simulink model "V2V"  (R2021a)
settings: Solver=FixedStepDiscrete  StartTime=0.0  StopTime=10  FixedStep=0.001  RelTol=1e-3
settings Model: Creator=maurizio  LastModifiedBy=maurizio
settings SolverCC: MinimalZcImpactIntegration=on
settings DebuggingCC: ReadBeforeWriteMsg=DisableAll  WriteAfterWriteMsg=DisableAll  WriteAfterReadMsg=DisableAll  MultiTaskDSMMsg=none  UnconnectedInputMsg=none  UnconnectedOutputMsg=none  UnconnectedLineMsg=none
settings ModelReferenceCC: UpdateModelReferenceTargets=IfOutOfDate  EnableRefExpFcnMdlSchedulingChecks=off
settings SFSimCC: SFSimEcho=off
settings RTWCC: Description=Generic Real-Time Target  BuildConfiguration=Faster Runs  DLArmComputeVersion=20.02.1

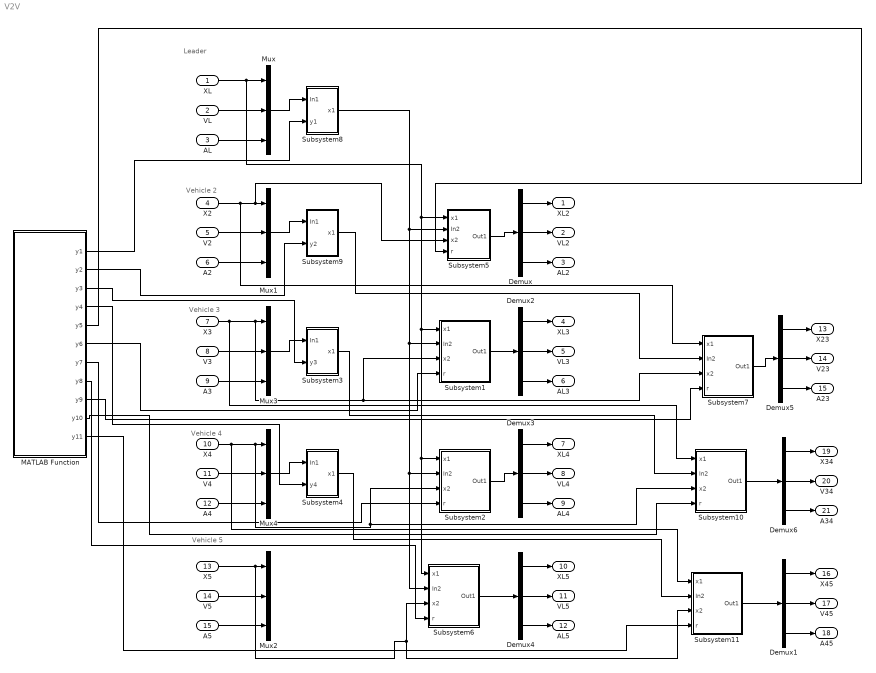
== system V2V ==
  note: Vehicle 3
  note: Vehicle 5
  note: Vehicle 4
  note: Vehicle 2
  note: Leader
  XL : Inport
  VL : Inport  Port=2
  AL : Inport  Port=3
  X2 : Inport  Port=4
  V2 : Inport  Port=5
  A2 : Inport  Port=6
  X3 : Inport  Port=7
  V3 : Inport  Port=8
  A3 : Inport  Port=9
  X4 : Inport  Port=10
  V4 : Inport  Port=11
  A4 : Inport  Port=12
  X5 : Inport  Port=13
  V5 : Inport  Port=14
  A5 : Inport  Port=15
  Demux{,1..6} (7 alike) : Demux  Outputs=3
  MATLAB Function : MATLAB Function  TreatAsAtomicUnit=on  SystemSampleTime=0.1
  Mux{,1..4} (5 alike) : Mux  Inputs=3
  Subsystem1 : Subsystem
  Subsystem10 : Subsystem
  Subsystem11 : Subsystem
  Subsystem2 : Subsystem
  Subsystem3 : Subsystem
  Subsystem4 : Subsystem
  Subsystem5 : Subsystem
  Subsystem6 : Subsystem
  Subsystem7 : Subsystem
  Subsystem8 : Subsystem
  Subsystem9 : Subsystem
  XL2 : Outport
  VL2 : Outport  Port=2
  AL2 : Outport  Port=3
  XL3 : Outport  Port=4
  VL3 : Outport  Port=5
  AL3 : Outport  Port=6
  XL4 : Outport  Port=7
  VL4 : Outport  Port=8
  AL4 : Outport  Port=9
  XL5 : Outport  Port=10
  VL5 : Outport  Port=11
  AL5 : Outport  Port=12
  X23 : Outport  Port=13
  V23 : Outport  Port=14
  A23 : Outport  Port=15
  X45 : Outport  Port=16
  V45 : Outport  Port=17
  A45 : Outport  Port=18
  X34 : Outport  Port=19
  V34 : Outport  Port=20
  A34 : Outport  Port=21
  wires:
  VL/1 -> Mux/2
  XL/1 -> Subsystem5/1(x1), Subsystem6/1(x1), Subsystem2/1(x1), Subsystem1/1(x1), Mux/1
  AL/1 -> Mux/3
  X2/1 -> Subsystem7/1(x1), Subsystem5/3(x2), Mux1/1
  V2/1 -> Mux1/2
  A2/1 -> Mux1/3
  A3/1 -> Mux3/3
  V3/1 -> Mux3/2
  X4/1 -> Subsystem11/1(x1), Subsystem10/3(x2), Subsystem2/3(x2), Mux4/1
  A4/1 -> Mux4/3
  X3/1 -> Subsystem10/1(x1), Subsystem7/3(x2), Subsystem1/3(x2), Mux3/1
  V4/1 -> Mux4/2
  Demux/1 -> XL2/1
  Demux/2 -> VL2/1
  Demux/3 -> AL2/1
  Demux2/1 -> XL3/1
  Demux2/3 -> AL3/1
  Demux2/2 -> VL3/1
  Demux3/3 -> AL4/1
  Demux3/1 -> XL4/1
  Demux3/2 -> VL4/1
  Demux4/2 -> VL5/1
  Demux4/1 -> XL5/1
  Demux4/3 -> AL5/1
  Demux5/3 -> A23/1
  Demux5/2 -> V23/1
  Demux5/1 -> X23/1
  Demux1/3 -> A45/1
  Demux1/2 -> V45/1
  Demux1/1 -> X45/1
  Demux6/3 -> A34/1
  Demux6/2 -> V34/1
  Demux6/1 -> X34/1
  Mux1/1 -> Subsystem9/1(In1)
  Mux3/1 -> Subsystem3/1(In1)
  Mux4/1 -> Subsystem4/1(In1)
  Subsystem5/1(Out1) -> Demux/1
  Mux/1 -> Subsystem8/1(In1)
  Subsystem8/1(x1) -> Subsystem6/2(In2), Subsystem2/2(In2), Subsystem1/2(In2), Subsystem5/2(In2)
  Subsystem2/1(Out1) -> Demux3/1
  Subsystem6/1(Out1) -> Demux4/1
  V5/1 -> Mux2/2
  A5/1 -> Mux2/3
  X5/1 -> Subsystem11/3(x2), Subsystem6/3(x2), Mux2/1
  Subsystem1/1(Out1) -> Demux2/1
  Subsystem7/1(Out1) -> Demux5/1
  Subsystem10/1(Out1) -> Demux6/1
  Subsystem11/1(Out1) -> Demux1/1
  Subsystem9/1(x1) -> Subsystem7/2(In2)
  Subsystem3/1(x1) -> Subsystem10/2(In2)
  Subsystem4/1(x1) -> Subsystem11/2(In2)
  MATLAB Function/1(y1) -> Subsystem8/2(y1)
  MATLAB Function/2(y2) -> Subsystem9/2(y2)
  MATLAB Function/3(y3) -> Subsystem3/2(y3)
  MATLAB Function/4(y4) -> Subsystem4/2(y4)
  MATLAB Function/5(y5) -> Subsystem5/4(r)
  MATLAB Function/6(y6) -> Subsystem1/4(r)
  MATLAB Function/7(y7) -> Subsystem2/4(r)
  MATLAB Function/8(y8) -> Subsystem6/4(r)
  MATLAB Function/9(y9) -> Subsystem7/4(r)
  MATLAB Function/10(y10) -> Subsystem10/4(r)
  MATLAB Function/11(y11) -> Subsystem11/4(r)

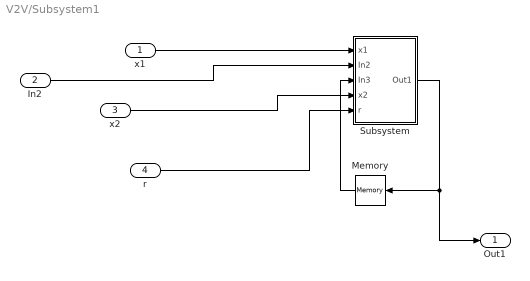
== system V2V/Subsystem1 ==
  x1 : Inport
  In2 : Inport  Port=2
  x2 : Inport  Port=3
  r : Inport  Port=4
  Memory : Memory
  Subsystem : Subsystem
  Out1 : Outport
  wires:
  Memory/1 -> Subsystem/3(In3)
  x2/1 -> Subsystem/4(x2)
  Subsystem/1(Out1) -> Out1/1, Memory/1
  x1/1 -> Subsystem/1(x1)
  In2/1 -> Subsystem/2(In2)
  r/1 -> Subsystem/5(r)

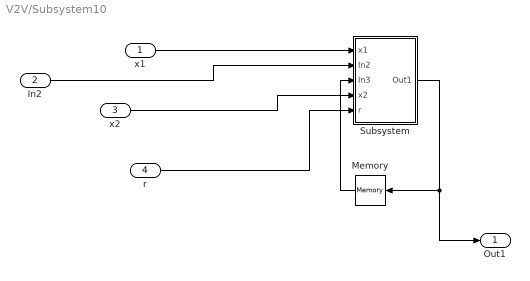
== system V2V/Subsystem10 ==
  x1 : Inport
  In2 : Inport  Port=2
  x2 : Inport  Port=3
  r : Inport  Port=4
  Memory : Memory
  Subsystem : Subsystem
  Out1 : Outport
  wires:
  Memory/1 -> Subsystem/3(In3)
  x2/1 -> Subsystem/4(x2)
  Subsystem/1(Out1) -> Out1/1, Memory/1
  x1/1 -> Subsystem/1(x1)
  In2/1 -> Subsystem/2(In2)
  r/1 -> Subsystem/5(r)

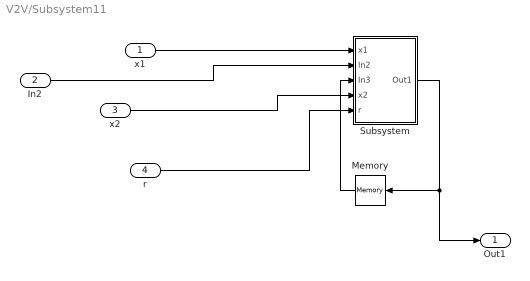
== system V2V/Subsystem11 ==
  x1 : Inport
  In2 : Inport  Port=2
  x2 : Inport  Port=3
  r : Inport  Port=4
  Memory : Memory
  Subsystem : Subsystem
  Out1 : Outport
  wires:
  Memory/1 -> Subsystem/3(In3)
  x2/1 -> Subsystem/4(x2)
  Subsystem/1(Out1) -> Out1/1, Memory/1
  x1/1 -> Subsystem/1(x1)
  In2/1 -> Subsystem/2(In2)
  r/1 -> Subsystem/5(r)

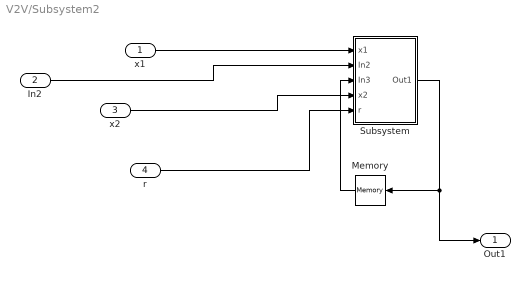
== system V2V/Subsystem2 ==
  x1 : Inport
  In2 : Inport  Port=2
  x2 : Inport  Port=3
  r : Inport  Port=4
  Memory : Memory
  Subsystem : Subsystem
  Out1 : Outport
  wires:
  Memory/1 -> Subsystem/3(In3)
  x2/1 -> Subsystem/4(x2)
  Subsystem/1(Out1) -> Out1/1, Memory/1
  x1/1 -> Subsystem/1(x1)
  In2/1 -> Subsystem/2(In2)
  r/1 -> Subsystem/5(r)

== system V2V/Subsystem3 ==
  In1 : Inport
  y3 : Inport  Port=2
  Delay : Delay  DelayLengthSource=Input port  DelayLengthUpperLimit=1000  SampleTime=0.001
      settings: InputPortMap=u0,p1
  Rate Transition1 : RateTransition  OutPortSampleTimeMultiple=100  OutPortSampleTime=0.1
  x1 : Outport
  wires:
  y3/1 -> Delay/2
  Rate Transition1/1 -> Delay/1
  Delay/1 -> x1/1
  In1/1 -> Rate Transition1/1

== system V2V/Subsystem4 ==
  In1 : Inport
  y4 : Inport  Port=2
  Delay : Delay  DelayLengthSource=Input port  DelayLengthUpperLimit=1000  SampleTime=0.001
      settings: InputPortMap=u0,p1
  Rate Transition1 : RateTransition  OutPortSampleTimeMultiple=100  OutPortSampleTime=0.1
  x1 : Outport
  wires:
  y4/1 -> Delay/2
  Rate Transition1/1 -> Delay/1
  Delay/1 -> x1/1
  In1/1 -> Rate Transition1/1

== system V2V/Subsystem5 ==
  x1 : Inport
  In2 : Inport  Port=2
  x2 : Inport  Port=3
  r : Inport  Port=4
  Memory : Memory
  Subsystem : Subsystem
  Out1 : Outport
  wires:
  Memory/1 -> Subsystem/3(In3)
  x2/1 -> Subsystem/4(x2)
  Subsystem/1(Out1) -> Out1/1, Memory/1
  x1/1 -> Subsystem/1(x1)
  In2/1 -> Subsystem/2(In2)
  r/1 -> Subsystem/5(r)

== system V2V/Subsystem6 ==
  x1 : Inport
  In2 : Inport  Port=2
  x2 : Inport  Port=3
  r : Inport  Port=4
  Memory : Memory
  Subsystem : Subsystem
  Out1 : Outport
  wires:
  Memory/1 -> Subsystem/3(In3)
  x2/1 -> Subsystem/4(x2)
  Subsystem/1(Out1) -> Out1/1, Memory/1
  x1/1 -> Subsystem/1(x1)
  In2/1 -> Subsystem/2(In2)
  r/1 -> Subsystem/5(r)

== system V2V/Subsystem7 ==
  x1 : Inport
  In2 : Inport  Port=2
  x2 : Inport  Port=3
  r : Inport  Port=4
  Memory : Memory
  Subsystem : Subsystem
  Out1 : Outport
  wires:
  Memory/1 -> Subsystem/3(In3)
  x2/1 -> Subsystem/4(x2)
  Subsystem/1(Out1) -> Out1/1, Memory/1
  x1/1 -> Subsystem/1(x1)
  In2/1 -> Subsystem/2(In2)
  r/1 -> Subsystem/5(r)

== system V2V/Subsystem8 ==
  In1 : Inport
  y1 : Inport  Port=2
  Delay : Delay  DelayLengthSource=Input port  DelayLengthUpperLimit=1000  SampleTime=0.001
      settings: InputPortMap=u0,p1
  Rate Transition1 : RateTransition  OutPortSampleTimeMultiple=100  OutPortSampleTime=0.1
  x1 : Outport
  wires:
  y1/1 -> Delay/2
  Rate Transition1/1 -> Delay/1
  Delay/1 -> x1/1
  In1/1 -> Rate Transition1/1

== system V2V/Subsystem9 ==
  In1 : Inport
  y2 : Inport  Port=2
  Delay : Delay  DelayLengthSource=Input port  DelayLengthUpperLimit=1000  SampleTime=0.001
      settings: InputPortMap=u0,p1
  Rate Transition1 : RateTransition  OutPortSampleTimeMultiple=100  OutPortSampleTime=0.1
  x1 : Outport
  wires:
  y2/1 -> Delay/2
  Rate Transition1/1 -> Delay/1
  Delay/1 -> x1/1
  In1/1 -> Rate Transition1/1

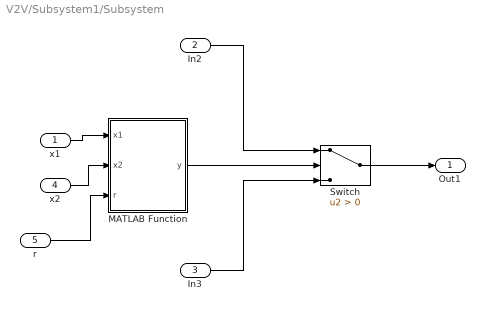
== system V2V/Subsystem1/Subsystem ==
  x1 : Inport
  In2 : Inport  Port=2
  In3 : Inport  Port=3
  x2 : Inport  Port=4
  r : Inport  Port=5
  MATLAB Function : MATLAB Function  TreatAsAtomicUnit=on  SystemSampleTime=0.1
  Switch : Switch  Criteria=u2 > Threshold
  Out1 : Outport
  wires:
  x2/1 -> MATLAB Function/2(x2)
  x1/1 -> MATLAB Function/1(x1)
  Switch/1 -> Out1/1
  In2/1 -> Switch/1
  In3/1 -> Switch/3
  MATLAB Function/1(y) -> Switch/2
  r/1 -> MATLAB Function/3(r)

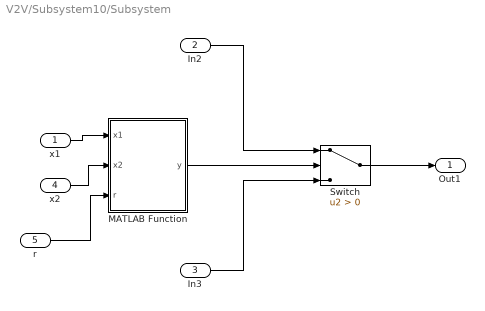
== system V2V/Subsystem10/Subsystem ==
  x1 : Inport
  In2 : Inport  Port=2
  In3 : Inport  Port=3
  x2 : Inport  Port=4
  r : Inport  Port=5
  MATLAB Function : MATLAB Function  TreatAsAtomicUnit=on  SystemSampleTime=0.1
  Switch : Switch  Criteria=u2 > Threshold
  Out1 : Outport
  wires:
  x2/1 -> MATLAB Function/2(x2)
  x1/1 -> MATLAB Function/1(x1)
  Switch/1 -> Out1/1
  In2/1 -> Switch/1
  In3/1 -> Switch/3
  MATLAB Function/1(y) -> Switch/2
  r/1 -> MATLAB Function/3(r)

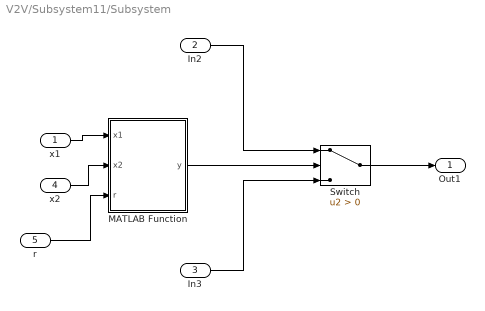
== system V2V/Subsystem11/Subsystem ==
  x1 : Inport
  In2 : Inport  Port=2
  In3 : Inport  Port=3
  x2 : Inport  Port=4
  r : Inport  Port=5
  MATLAB Function : MATLAB Function  TreatAsAtomicUnit=on  SystemSampleTime=0.1
  Switch : Switch  Criteria=u2 > Threshold
  Out1 : Outport
  wires:
  x2/1 -> MATLAB Function/2(x2)
  x1/1 -> MATLAB Function/1(x1)
  Switch/1 -> Out1/1
  In2/1 -> Switch/1
  In3/1 -> Switch/3
  MATLAB Function/1(y) -> Switch/2
  r/1 -> MATLAB Function/3(r)

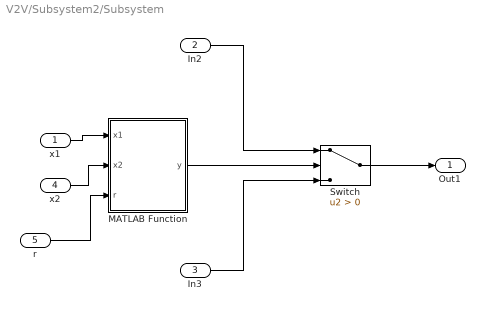
== system V2V/Subsystem2/Subsystem ==
  x1 : Inport
  In2 : Inport  Port=2
  In3 : Inport  Port=3
  x2 : Inport  Port=4
  r : Inport  Port=5
  MATLAB Function : MATLAB Function  TreatAsAtomicUnit=on  SystemSampleTime=0.1
  Switch : Switch  Criteria=u2 > Threshold
  Out1 : Outport
  wires:
  x2/1 -> MATLAB Function/2(x2)
  x1/1 -> MATLAB Function/1(x1)
  Switch/1 -> Out1/1
  In2/1 -> Switch/1
  In3/1 -> Switch/3
  MATLAB Function/1(y) -> Switch/2
  r/1 -> MATLAB Function/3(r)

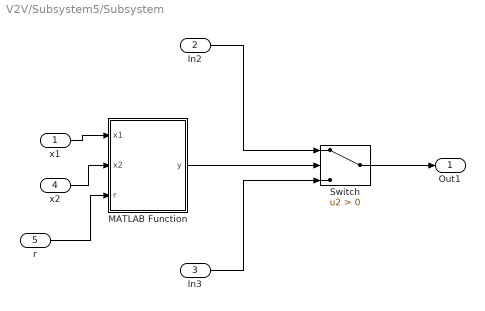
== system V2V/Subsystem5/Subsystem ==
  x1 : Inport
  In2 : Inport  Port=2
  In3 : Inport  Port=3
  x2 : Inport  Port=4
  r : Inport  Port=5
  MATLAB Function : MATLAB Function  TreatAsAtomicUnit=on  SystemSampleTime=0.1
  Switch : Switch  Criteria=u2 > Threshold
  Out1 : Outport
  wires:
  x2/1 -> MATLAB Function/2(x2)
  x1/1 -> MATLAB Function/1(x1)
  Switch/1 -> Out1/1
  In2/1 -> Switch/1
  In3/1 -> Switch/3
  MATLAB Function/1(y) -> Switch/2
  r/1 -> MATLAB Function/3(r)

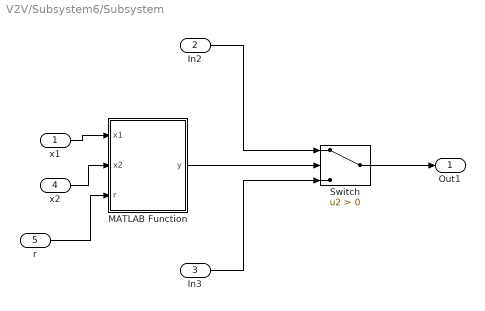
== system V2V/Subsystem6/Subsystem ==
  x1 : Inport
  In2 : Inport  Port=2
  In3 : Inport  Port=3
  x2 : Inport  Port=4
  r : Inport  Port=5
  MATLAB Function : MATLAB Function  TreatAsAtomicUnit=on  SystemSampleTime=0.1
  Switch : Switch  Criteria=u2 > Threshold
  Out1 : Outport
  wires:
  x2/1 -> MATLAB Function/2(x2)
  x1/1 -> MATLAB Function/1(x1)
  Switch/1 -> Out1/1
  In2/1 -> Switch/1
  In3/1 -> Switch/3
  MATLAB Function/1(y) -> Switch/2
  r/1 -> MATLAB Function/3(r)

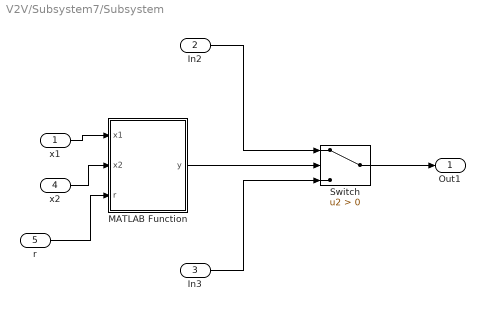
== system V2V/Subsystem7/Subsystem ==
  x1 : Inport
  In2 : Inport  Port=2
  In3 : Inport  Port=3
  x2 : Inport  Port=4
  r : Inport  Port=5
  MATLAB Function : MATLAB Function  TreatAsAtomicUnit=on  SystemSampleTime=0.1
  Switch : Switch  Criteria=u2 > Threshold
  Out1 : Outport
  wires:
  x2/1 -> MATLAB Function/2(x2)
  x1/1 -> MATLAB Function/1(x1)
  Switch/1 -> Out1/1
  In2/1 -> Switch/1
  In3/1 -> Switch/3
  MATLAB Function/1(y) -> Switch/2
  r/1 -> MATLAB Function/3(r)

== matlab function V2V/Subsystem1/Subsystem/MATLAB Function ==
  data: x1 input; y output; x2 input; r input
function y = fcn(x1,x2,r)
    PDR = model80211p(0.12,25,23,190,6e6,x1-x2);

    y = r < PDR;
end

== matlab function V2V/Subsystem2/Subsystem/MATLAB Function ==
  data: x1 input; y output; x2 input; r input
function y = fcn(x1,x2,r)
    PDR = model80211p(0.12,25,23,190,6e6,x1-x2);

    y = r < PDR;
end

== matlab function V2V/Subsystem6/Subsystem/MATLAB Function ==
  data: x1 input; y output; x2 input; r input
function y = fcn(x1,x2,r)
    PDR = model80211p(0.12,25,23,190,6e6,x1-x2);

    y = r < PDR;
end

== matlab function V2V/Subsystem7/Subsystem/MATLAB Function ==
  data: x1 input; y output; x2 input; r input
function y = fcn(x1,x2,r)
    PDR = model80211p(0.12,25,23,190,6e6,x1-x2);

    y = r < PDR;
end

== matlab function V2V/MATLAB Function ==
  data: y1 output; y2 output; y3 output; y4 output; y5 output; y6 output; y7 output; y8 output; y9 output; y10 output; y11 output
function [y1,y2,y3,y4,y5,y6,y7,y8, y9,y10,y11] = fcn
y1 = ceil(exprnd(20));
y2 = ceil(exprnd(20));
y3 = ceil(exprnd(20));
y4 = ceil(exprnd(20));
y5 = rand;
y6 = rand;
y7 = rand;
y8 = rand;
y9 = rand;
y10 = rand;
y11 = rand;
end

== matlab function V2V/Subsystem10/Subsystem/MATLAB Function ==
  data: x1 input; y output; x2 input; r input
function y = fcn(x1,x2,r)
    PDR = model80211p(0.12,25,23,190,6e6,x1-x2);

    y = r < PDR;
end

== matlab function V2V/Subsystem11/Subsystem/MATLAB Function ==
  data: x1 input; y output; x2 input; r input
function y = fcn(x1,x2,r)
    PDR = model80211p(0.12,25,23,190,6e6,x1-x2);

    y = r < PDR;
end

== matlab function V2V/Subsystem5/Subsystem/MATLAB Function ==
  data: x1 input; y output; x2 input; r input
function y = fcn(x1,x2,r)
    PDR = model80211p(0.12,25,23,190,6e6,x1-x2);

    y = r < PDR;
end
